simulink model "continuousanddiscretecontrol"  (R2013b)
settings: Solver=ode45  StartTime=0.0  StopTime=10.0  RelTol=1e-3
undefined symbols (not defined in the file): a, b, c, d, K, m, n, p, q, r
settings Model: Creator=tvincent  LastModifiedBy=tvincent

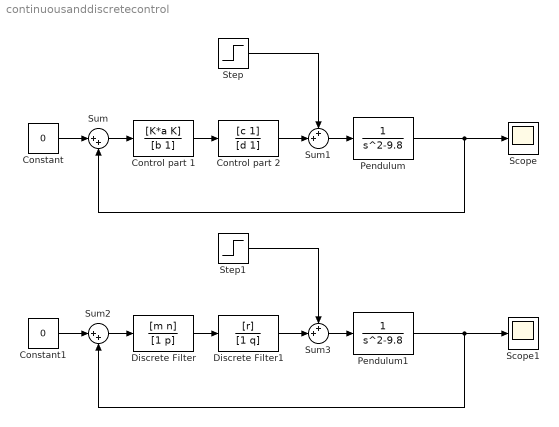
== system continuousanddiscretecontrol ==
  Constant : Constant  Value=0
  Constant1 : Constant  Value=0
  Control part 1 : TransferFcn  Numerator=[K*a K]  Denominator=[b 1]
  Control part 2 : TransferFcn  Numerator=[c 1]  Denominator=[d 1]
  Discrete Filter : DiscreteFilter  Numerator=[m n]  Denominator=[1 p]
  Discrete Filter1 : DiscreteFilter  Numerator=[r]  Denominator=[1 q]
  Pendulum : TransferFcn  Denominator=[1 0 -9.8]
  Pendulum1 : TransferFcn  Denominator=[1 0 -9.8]
  Scope : Scope
  Scope1 : Scope
  Step : Step  SampleTime=0
  Step1 : Step  SampleTime=0
  Sum : Sum  Inputs=|++
  Sum1 : Sum  Inputs=++|
  Sum2 : Sum  Inputs=|++
  Sum3 : Sum  Inputs=++|
  wires:
  Pendulum/1 -> Sum/2, Scope/1
  Sum/1 -> Control part 1/1
  Constant/1 -> Sum/1
  Sum1/1 -> Pendulum/1
  Step/1 -> Sum1/1
  Control part 1/1 -> Control part 2/1
  Control part 2/1 -> Sum1/2
  Pendulum1/1 -> Sum2/2, Scope1/1
  Sum2/1 -> Discrete Filter/1
  Constant1/1 -> Sum2/1
  Sum3/1 -> Pendulum1/1
  Step1/1 -> Sum3/1
  Discrete Filter/1 -> Discrete Filter1/1
  Discrete Filter1/1 -> Sum3/2
